simulink model "DragModelAIAAv3"  (R2018b)
settings: Solver=VariableStepAuto  StartTime=0.0  StopTime=10.0  RelTol=1e-3  EnableMultiTasking=on
undefined symbols (not defined in the file): Aero, Uav
settings Model: Creator=jban039  LastModifiedBy=jban039
settings DataIOCC: LimitDataPoints=on
settings OptimizationCC: LifeSpan=inf
settings DebuggingCC: AllowSymbolicDim=off  SFUnexpectedBacktrackingDiag=warning  SFNoUnconditionalDefaultTransitionDiag=warning  SFExecutionAtInitializationDiag=none
settings ModelReferenceCC: PropagateSignalLabelsOutOfModel=off
settings SFSimCC: SimUseLocalCustomCode=off
settings RTWCC: RTWUseLocalCustomCode=off
settings CodeAppCC: StateflowObjectComments=on
settings GRTTargetCC: TargetLangStandard=C89/C90 (ANSI)
settings ConfigComp: CovMetricSettings=dw  CovHtmlReporting=on  CovSaveCumulativeToWorkspaceVar=on  CovSaveSingleToWorkspaceVar=on  CovExternalEMLEnable=off

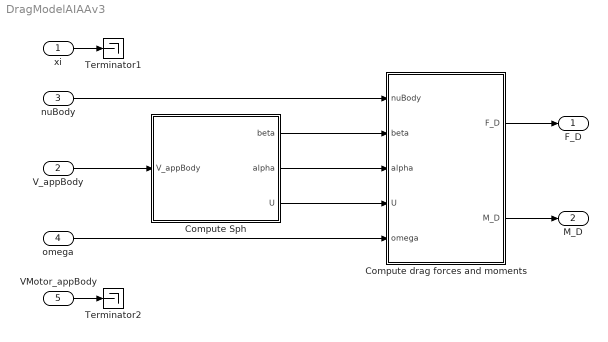
== system DragModelAIAAv3 ==
  xi : Inport  Unit=m  PortDimensions=3
  V_appBody : Inport  Port=2  Unit=m/s  PortDimensions=3
  nuBody : Inport  Port=3  Unit=rad/s  PortDimensions=3
  omega : Inport  Port=4  Unit=rad/s  PortDimensions=Uav.N_ROTORS
  VMotor_appBody : Inport  Port=5  Unit=m/s  PortDimensions=[3,Uav.N_ROTORS]
  Compute Sph : MATLAB Function  TreatAsAtomicUnit=on
  Compute drag forces and moments : MATLAB Function  TreatAsAtomicUnit=on
  Terminator1 : Terminator
  Terminator2 : Terminator
  F_D : Outport  Unit=N
  M_D : Outport  Port=2  Unit=N*m
  wires:
  Compute drag forces and moments/1(F_D) -> F_D/1
  xi/1 -> Terminator1/1
  omega/1 -> Compute drag forces and moments/5(omega)
  nuBody/1 -> Compute drag forces and moments/1(nuBody)
  Compute Sph/3(U) -> Compute drag forces and moments/4(U)
  Compute Sph/2(alpha) -> Compute drag forces and moments/3(alpha)
  Compute Sph/1(beta) -> Compute drag forces and moments/2(beta)
  VMotor_appBody/1 -> Terminator2/1
  Compute drag forces and moments/2(M_D) -> M_D/1
  V_appBody/1 -> Compute Sph/1(V_appBody)

== matlab function DragModelAIAAv3/Compute Sph ==
  data: V_appBody input; beta output; alpha output; U output
function [beta, alpha, U] = computeSph(V_appBody)
%#codegen

% Convert from polar to spherical coordinates
[ beta, alpha, U ] = cart2sph( V_appBody(1), V_appBody(2), V_appBody(3) );

== matlab function DragModelAIAAv3/Compute drag forces and moments ==
  data: nuBody input; beta input; alpha input; U input; omega input; F_D output; M_D output; Uav parameter; Aero parameter
function [F_D, M_D] = computeDrag( nuBody, beta, alpha, U, ...
                                   omega, Uav, Aero )
%#codegen
% Outputs
F_D = zeros(3,1);
M_D = zeros(3,1);

% Forces
Cz1 = dot( Aero.Cz1.coefs, [sin(alpha), 1] );
Cx1 = dot( Aero.Cx1.coefs, [cos(alpha), cos(3*alpha), cos(7*alpha)] );
faero_z = -0.5 .* Uav.RHO_AIR .* U^2 .* Cz1 * Uav.A_UAV;
faero_x = -0.5 .* Uav.RHO_AIR .* U^2 .* Cx1 * Uav.A_UAV;
F_D = [faero_x*cos(beta); faero_x*sin(beta); faero_z];

% Moments
CM1 = dot( Aero.CM1.coefs, [cos(alpha), cos(3*alpha), sin(2*alpha)] );
p = Aero.CM2.coefs;
lambda = omega .* Uav.D_PROP / ( 2 * U );
CM2 = p(1) .* ( 1 - exp(-p(2).*lambda) ) .* cos(alpha) + ...
      p(3) .* ( 1 - exp(-p(4).*lambda) ) .* sin(2*alpha);
m_D = 0.5 .* Uav.RHO_AIR .* U^2 * CM1 * Uav.A_UAV .* Uav.D_UAV + ...
      0.5 .* Uav.RHO_AIR .* U * sum(omega .* CM2) .* Uav.A_PROP .* Uav.D_PROP^2;
M_D = [ -sin(beta)*m_D; cos(beta)*m_D; 0 ];
